simulink model "test_leds"  (R2013a)
settings: Solver=FixedStepDiscrete  StartTime=0.0  StopTime=5  FixedStep=0.1  RelTol=1e-3
libraries: ardrone_lib x4
settings Model: Creator=Arnaud  LastModifiedBy=Arnaud
settings OptimizationCC: InitFltsAndDblsToZero=on  OptimizeModelRefInitCode=on  LifeSpan=1
settings RTWCC: SystemTargetFile=ardrone.tlc  TemplateMakefile=ardrone.tmf  Description=AR.Drone_v2  ProcessScript=ardrone_make_rtw_hook  TargetLang=C++
settings CodeAppCC: IgnoreCustomStorageClasses=off
settings STFCustomTargetCC: GenerateSampleERTMain=on  ModelReferenceCompliant=off  CombineOutputUpdateFcns=on  ERTCustomFileBanners=on  SupportContinuousTime=off  SupportNonInlinedSFcns=off  MATLABClassNameForMDSCustomization=Simulink.SoftwareTarget.ERTCustomization  SystemTargetFile=ardrone.tlc
settings ERTTargetCC: ModelReferenceCompliant=off  ParMdlRefBuildCompliant=off  CompOptLevelCompliant=off  ConcurrentExecutionCompliant=off  ERTFirstTimeCompliant=off  ModelStepFunctionPrototypeControlCompliant=off  CPPClassGenCompliant=off  InlinedParameterPlacement=Hierarchical  ERTSrcFileBannerTemplate=example_banner.tlc  ERTHdrFileBannerTemplate=example_banner.tlc  ERTCustomFileTemplate=ardrone_file_process.tlc

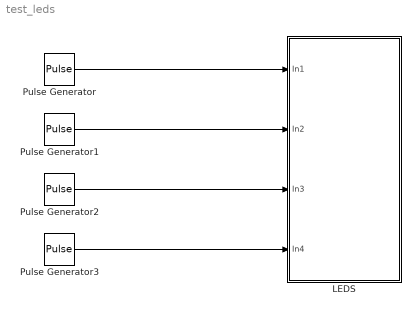
== system test_leds ==
  LEDS : Subsystem
  Pulse Generator : DiscretePulseGenerator  PulseType=Time based  Period=0.6  PulseWidth=50
  Pulse Generator1 : DiscretePulseGenerator  PulseType=Time based  Amplitude=2  Period=0.6  PulseWidth=50
  Pulse Generator2 : DiscretePulseGenerator  PulseType=Time based  Period=1.2  PulseWidth=50
  Pulse Generator3 : DiscretePulseGenerator  PulseType=Time based  Amplitude=2  Period=1.2  PulseWidth=50
  wires:
  Pulse Generator/1 -> LEDS/1(In1)
  Pulse Generator1/1 -> LEDS/2(In2)
  Pulse Generator2/1 -> LEDS/3(In3)
  Pulse Generator3/1 -> LEDS/4(In4)

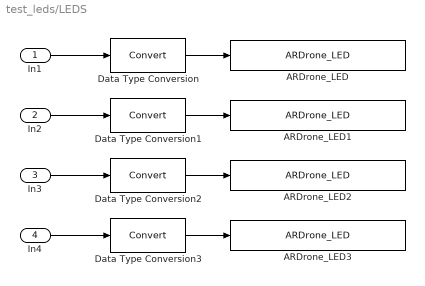
== system test_leds/LEDS ==
  In1 : Inport
  In2 : Inport  Port=2
  In3 : Inport  Port=3
  In4 : Inport  Port=4
  ARDrone_LED : ardrone_lib/ARDrone_LED  SFunctionSpec=void LED_Set(int32 u1, uint8 p1)  SParameter1=0  ShowSpec=on
  ARDrone_LED1 : ardrone_lib/ARDrone_LED  SFunctionSpec=void LED_Set(int32 u1, uint8 p1)  SParameter1=1  ShowSpec=on
  ARDrone_LED2 : ardrone_lib/ARDrone_LED  SFunctionSpec=void LED_Set(int32 u1, uint8 p1)  SParameter1=2  ShowSpec=on
  ARDrone_LED3 : ardrone_lib/ARDrone_LED  SFunctionSpec=void LED_Set(int32 u1, uint8 p1)  SParameter1=3  ShowSpec=on
  Data Type Conversion{,1..3} (4 alike) : DataTypeConversion
  wires:
  In1/1 -> Data Type Conversion/1
  In2/1 -> Data Type Conversion1/1
  In3/1 -> Data Type Conversion2/1
  In4/1 -> Data Type Conversion3/1
  Data Type Conversion3/1 -> ARDrone_LED3/1
  Data Type Conversion1/1 -> ARDrone_LED1/1
  Data Type Conversion2/1 -> ARDrone_LED2/1
  Data Type Conversion/1 -> ARDrone_LED/1
